simulink model "III_phase_voltage_sourse_inverter"  (R2022a)
settings: Solver=VariableStepAuto  StartTime=0.0  StopTime=10.0  RelTol=1e-3
undefined symbols (not defined in the file): L, R, Vdc, w
settings Model: Creator=darsh  LastModifiedBy=darsh
settings ConfigComp: CovScope=ReferencedModels

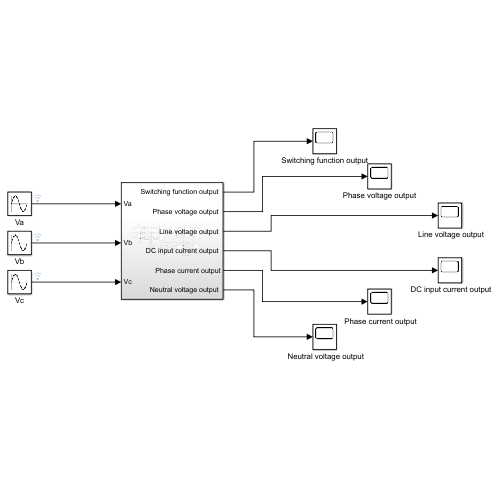
[thumbnail: Simulink's stored preview of the top-level diagram]
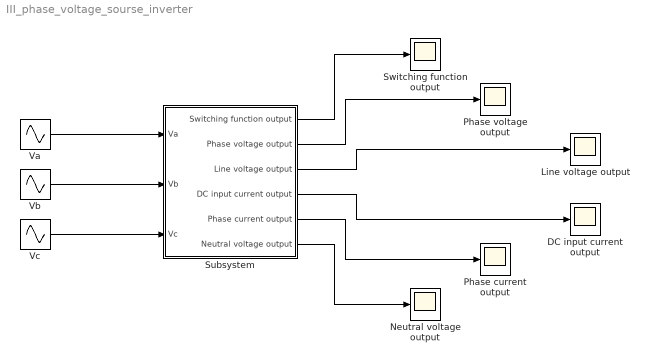
== system III_phase_voltage_sourse_inverter ==
  " DC input current output " : Scope
  " Line voltage output " : Scope
  " Neutral voltage output " : Scope
  " Phase current output" : Scope
  "Phase voltage output " : Scope
  Subsystem : Subsystem
  "Switching function output " : Scope
  Va : Sin  Frequency=2*pi*50  SampleTime=0
  Vb : Sin  Frequency=2*pi*50  Phase=-2*pi/3  SampleTime=0
  Vc : Sin  Frequency=2*pi*50  Phase=2*pi/3  SampleTime=0
  wires:
  Va/1 -> Subsystem/1(Va)
  Vb/1 -> Subsystem/2(Vb)
  Vc/1 -> Subsystem/3(Vc)
  Subsystem/1("Switching function output ") -> "Switching function output "/1
  Subsystem/2("Phase voltage output ") -> "Phase voltage output "/1
  Subsystem/3("Line voltage output ") -> " Line voltage output "/1
  Subsystem/4("DC input current output ") -> " DC input current output "/1
  Subsystem/5(Phase current output) -> " Phase current output"/1
  Subsystem/6("Neutral voltage output ") -> " Neutral voltage output "/1

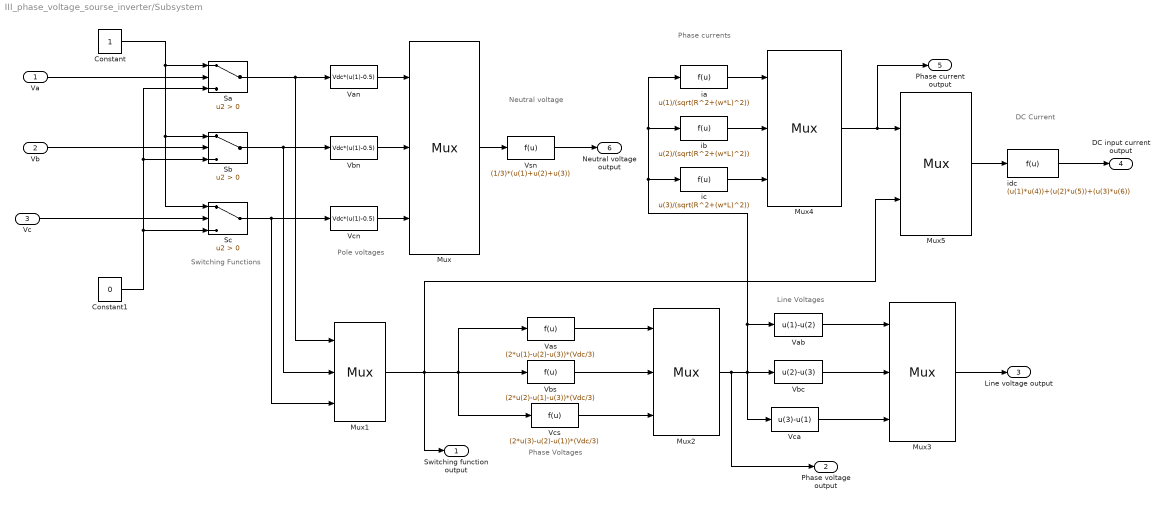
== system III_phase_voltage_sourse_inverter/Subsystem ==
  note: Neutral voltage
  note: Phase currents
  note: Pole voltages
  note: Switching Functions
  note: Line Voltages
  note: Phase Voltages
  note: DC Current
  Va : Inport
  Vb : Inport  Port=2
  Vc : Inport  Port=3
  Constant : Constant
  Constant1 : Constant  Value=0
  Mux{,1..4} (5 alike) : Mux  Inputs=3
  Mux5 : Mux  Inputs=2
  Sa : Switch  Criteria=u2 > Threshold  SaturateOnIntegerOverflow=off  InputSameDT=off
  Sb : Switch  Criteria=u2 > Threshold  SaturateOnIntegerOverflow=off  InputSameDT=off
  Sc : Switch  Criteria=u2 > Threshold  SaturateOnIntegerOverflow=off  InputSameDT=off
  Vab : Fcn  Expr=u(1)-u(2)
  Van : Fcn  Expr=Vdc*(u(1)-0.5)
  Vas : Fcn  Expr=(2*u(1)-u(2)-u(3))*(Vdc/3)
  Vbc : Fcn  Expr=u(2)-u(3)
  Vbn : Fcn  Expr=Vdc*(u(1)-0.5)
  Vbs : Fcn  Expr=(2*u(2)-u(1)-u(3))*(Vdc/3)
  Vca : Fcn  Expr=u(3)-u(1)
  Vcn : Fcn  Expr=Vdc*(u(1)-0.5)
  Vcs : Fcn  Expr=(2*u(3)-u(2)-u(1))*(Vdc/3)
  Vsn : Fcn  Expr=(1/3)*(u(1)+u(2)+u(3))
  ia : Fcn  Expr=u(1)/(sqrt(R^2+(w*L)^2))
  ib : Fcn  Expr=u(2)/(sqrt(R^2+(w*L)^2))
  ic : Fcn  Expr=u(3)/(sqrt(R^2+(w*L)^2))
  "idc " : Fcn  Expr=(u(1)*u(4))+(u(2)*u(5))+(u(3)*u(6))
  "Switching function output " : Outport  VectorParamsAs1DForOutWhenUnconnected=off
  "Phase voltage output " : Outport  Port=2  VectorParamsAs1DForOutWhenUnconnected=off
  "Line voltage output " : Outport  Port=3  VectorParamsAs1DForOutWhenUnconnected=off
  "DC input current output " : Outport  Port=4  VectorParamsAs1DForOutWhenUnconnected=off
  Phase current output : Outport  Port=5  VectorParamsAs1DForOutWhenUnconnected=off
  "Neutral voltage output " : Outport  Port=6  VectorParamsAs1DForOutWhenUnconnected=off
  wires:
  Constant1/1 -> Sa/3, Sb/3, Sc/3
  Vb/1 -> Sb/2
  Vcn/1 -> Mux/3
  Vbc/1 -> Mux3/2
  Mux1/1 -> "Switching function output "/1, Mux5/2, Vas/1, Vcs/1, Vbs/1
  Van/1 -> Mux/1
  "idc "/1 -> "DC input current output "/1
  Mux2/1 -> "Phase voltage output "/1, Vbc/1, Vca/1, Vab/1, ia/1, ib/1, ic/1
  Vbs/1 -> Mux2/2
  Mux4/1 -> Phase current output/1, Mux5/1
  Sc/1 -> Mux1/3, Vcn/1
  Vas/1 -> Mux2/1
  Mux5/1 -> "idc "/1
  Vab/1 -> Mux3/1
  Va/1 -> Sa/2
  ib/1 -> Mux4/2
  Sb/1 -> Mux1/2, Vbn/1
  Mux/1 -> Vsn/1
  Vbn/1 -> Mux/2
  Sa/1 -> Mux1/1, Van/1
  Vcs/1 -> Mux2/3
  Vsn/1 -> "Neutral voltage output "/1
  Constant/1 -> Sc/1, Sb/1, Sa/1
  Vca/1 -> Mux3/3
  ic/1 -> Mux4/3
  Mux3/1 -> "Line voltage output "/1
  ia/1 -> Mux4/1
  Vc/1 -> Sc/2
